simulink model "udp_sine_gen"  (R2026a)
settings: Solver=FixedStepDiscrete  StopTime=inf  FixedStep=0.1
undefined symbols (not defined in the file or in its folder): f, f2ee6846, vps
libraries: instrumentlib x3
settings Model: Creator=dsamarka  LastModifiedBy=dsamarka

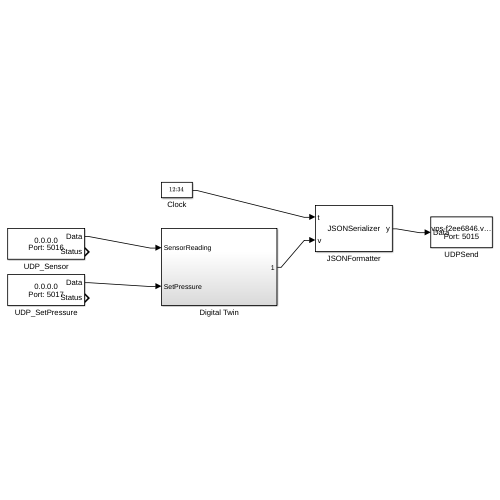
[thumbnail: Simulink's stored preview of the top-level diagram]
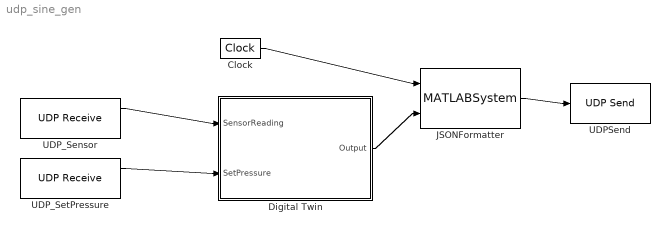
== system udp_sine_gen ==
  Clock : DigitalClock  SampleTime=0.1
  Digital Twin : Subsystem
  JSONFormatter : MATLABSystem  System=JSONSerializer  SimulateUsing=Code generation
      mask Type: JSONSerializer
  UDPSend : instrumentlib/UDP Send  Host=vps-f2ee6846.vps.ovh.net  Port=5015  LocalAddress=0.0.0.0  LocalPort=-1  EnablePortSharing=off  OutputDatagramPacketSize=512  ByteOrder=big-endian  EnableBlockingMode=on  SimulateUsing=Interpreted execution
  UDP_Sensor : instrumentlib/UDP Receive  LocalAddress=0.0.0.0  LocalPort=5016  EnablePortSharing=off  Host=localhost  Port=9090  GetLatestData=on  DataSize=1  DataType=double  ASCIIFormatting=%f,  Terminator=LF  CustomTerminator=10  ByteOrder=little-endian  EnableBlockingMode=off  Timeout=10  SampleTime=0.1  SimulateUsing=Interpreted execution
  UDP_SetPressure : instrumentlib/UDP Receive  LocalAddress=0.0.0.0  LocalPort=5017  EnablePortSharing=off  Host=localhost  Port=9090  GetLatestData=on  DataSize=1  DataType=double  ASCIIFormatting=%f,  Terminator=LF  CustomTerminator=10  ByteOrder=little-endian  EnableBlockingMode=off  Timeout=10  SampleTime=0.1  SimulateUsing=Interpreted execution
  wires:
  UDP_Sensor/1 -> Digital Twin/1(SensorReading)
  UDP_SetPressure/1 -> Digital Twin/2(SetPressure)
  Clock/1 -> JSONFormatter/1
  Digital Twin/1(Output) -> JSONFormatter/2
  JSONFormatter/1 -> UDPSend/1

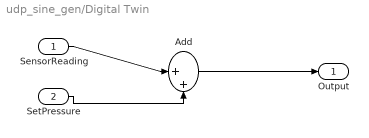
== system udp_sine_gen/Digital Twin ==
  SensorReading : Inport
  SetPressure : Inport  Port=2
  Add : Sum  Inputs=|++
  Output : Outport
  wires:
  SensorReading/1 -> Add/1
  SetPressure/1 -> Add/2
  Add/1 -> Output/1
